simulink model "avr"  (R2025a)
settings: Solver=VariableStepAuto  StartTime=0.0  StopTime=10.0  RelTol=1e-3
settings Model: Creator=Lijoofficial  LastModifiedBy=Lijoofficial

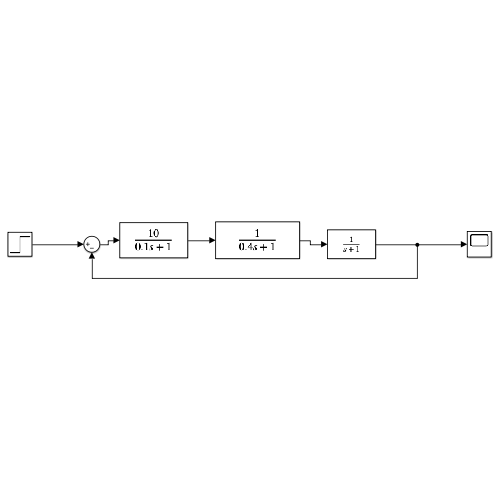
[thumbnail: Simulink's stored preview of the top-level diagram]
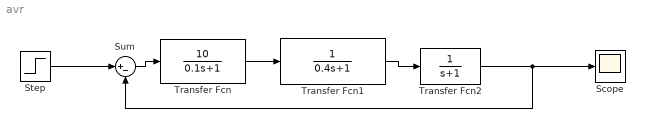
== system avr ==
  Scope : Scope
      settings: ActiveDisplayYMinimum=-0.183299404010295  ActiveDisplayYMaximum=1.6496946360926552
  Step : Step  Time=0  SampleTime=0
  Sum : Sum  Inputs=|+-
  Transfer Fcn : TransferFcn  Numerator=10  Denominator=[0.1 1]
  Transfer Fcn1 : TransferFcn  Denominator=[0.4 1]
  Transfer Fcn2 : TransferFcn  Denominator=[1 1]
  wires:
  Step/1 -> Sum/1
  Sum/1 -> Transfer Fcn/1
  Transfer Fcn/1 -> Transfer Fcn1/1
  Transfer Fcn1/1 -> Transfer Fcn2/1
  Transfer Fcn2/1 -> Sum/2, Scope/1
